simulink model "CluchLockUp"  (R2020b)
settings: Solver=VariableStepAuto  StartTime=0.0  StopTime=10.0  RelTol=1e-3
model workspace (MAT data in the model file):
  Fn = [0  0; 1  0.8; 2  1.6; 3  1.6; 4  1.6; 5  1.6; 6  0.8; 7  0; 8  0; 9  0; 10  0]
  Ie = 1
  Iv = 5
  R = 1
  Tin = [1  2; 2  2; 3  2; 4  2; 5  2; 6  0; 7  0; 8  0; 9  0; 10  0]
  be = 2
  bv = 1
  f1 = [1; 6; 11; 16; 21; 26; 31; 36; 41; 46; 51]
  muk = 1
  mus = 1.5
settings Model: Creator=baner  LastModifiedBy=baner

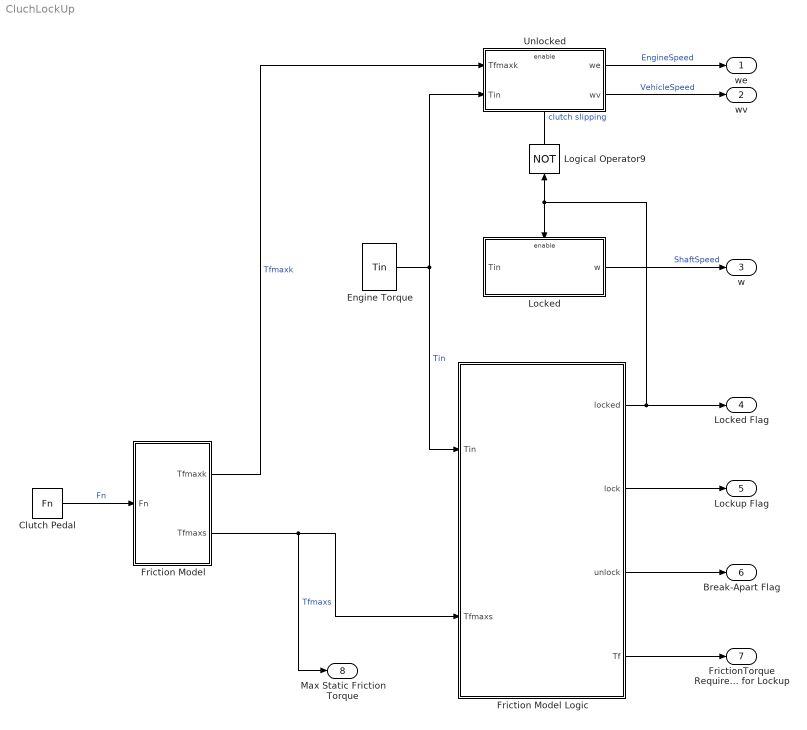
== system CluchLockUp ==
  Clutch Pedal : FromWorkspace  VariableName=Fn  ZeroCross=off
  Engine Torque : FromWorkspace  VariableName=Tin  ZeroCross=off
  Friction Model : Subsystem
  Friction Model Logic : Subsystem
  Locked : Subsystem  TreatAsAtomicUnit=on
  Logical Operator9 : Logic  Operator=NOT  Inputs=1  IconShape=distinctive  OutDataTypeStr=boolean
  Unlocked : Subsystem  TreatAsAtomicUnit=on
  we : Outport  InitialOutput=0  VectorParamsAs1DForOutWhenUnconnected=off
  wv : Outport  Port=2  InitialOutput=0  VectorParamsAs1DForOutWhenUnconnected=off
  w : Outport  Port=3  InitialOutput=0  VectorParamsAs1DForOutWhenUnconnected=off
  Locked Flag : Outport  Port=4  InitialOutput=0  VectorParamsAs1DForOutWhenUnconnected=off
  Lockup Flag : Outport  Port=5  InitialOutput=0  VectorParamsAs1DForOutWhenUnconnected=off
  Break-Apart Flag : Outport  Port=6  InitialOutput=0  VectorParamsAs1DForOutWhenUnconnected=off
  FrictionTorque Required for Lockup : Outport  Port=7  InitialOutput=0  VectorParamsAs1DForOutWhenUnconnected=off
  Max Static Friction Torque : Outport  Port=8  InitialOutput=0  VectorParamsAs1DForOutWhenUnconnected=off
  wires:
  Clutch Pedal/1 -> Friction Model/1(Fn)  "Fn"
  Logical Operator9/1 -> Unlocked/Enable  "clutch slipping"
  Friction Model Logic/1(locked) -> Logical Operator9/1, Locked/Enable, Locked Flag/1
  Engine Torque/1 -> Friction Model Logic/1(Tin), Unlocked/2(Tin)  "Tin"
  Friction Model/1(Tfmaxk) -> Unlocked/1(Tfmaxk)  "Tfmaxk"
  Friction Model/2(Tfmaxs) -> Max Static Friction Torque/1, Friction Model Logic/2(Tfmaxs)  "Tfmaxs"
  Unlocked/1(we) -> we/1  "EngineSpeed"
  Unlocked/2(wv) -> wv/1  "VehicleSpeed"
  Locked/1(w) -> w/1  "ShaftSpeed"
  Friction Model Logic/2(lock) -> Lockup Flag/1
  Friction Model Logic/3(unlock) -> Break-Apart Flag/1
  Friction Model Logic/4(Tf) -> FrictionTorque Required for Lockup/1

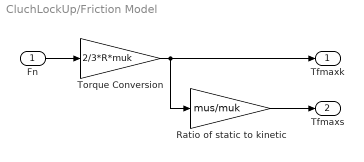
== system CluchLockUp/Friction Model ==
  Fn : Inport
  Ratio of static to kinetic : Gain  Gain=mus/muk  SaturateOnIntegerOverflow=on  OutDataTypeStr=Inherit: Same as input  ParamDataTypeStr=Inherit: Same as input
  Torque Conversion : Gain  Gain=2/3*R*muk  SaturateOnIntegerOverflow=on  OutDataTypeStr=Inherit: Same as input  ParamDataTypeStr=Inherit: Same as input
  Tfmaxk : Outport  InitialOutput=0  VectorParamsAs1DForOutWhenUnconnected=off
  Tfmaxs : Outport  Port=2  InitialOutput=0  VectorParamsAs1DForOutWhenUnconnected=off
  wires:
  Ratio of static to kinetic/1 -> Tfmaxs/1
  Fn/1 -> Torque Conversion/1
  Torque Conversion/1 -> Ratio of static to kinetic/1, Tfmaxk/1

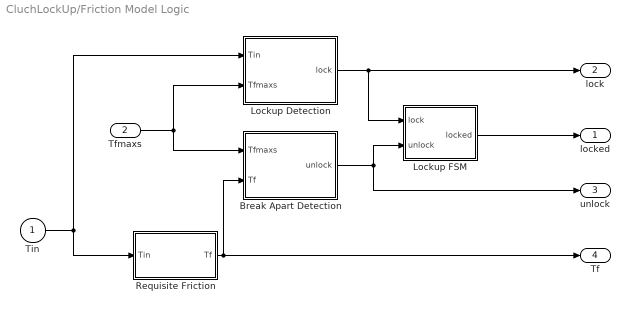
== system CluchLockUp/Friction Model Logic ==
  Tin : Inport
  Tfmaxs : Inport  Port=2
  Break Apart Detection : Subsystem
  Lockup Detection : Subsystem
  Lockup FSM : Subsystem
  Requisite Friction : Subsystem
  locked : Outport  InitialOutput=0  VectorParamsAs1DForOutWhenUnconnected=off
  lock : Outport  Port=2  InitialOutput=0  VectorParamsAs1DForOutWhenUnconnected=off
  unlock : Outport  Port=3  InitialOutput=0  VectorParamsAs1DForOutWhenUnconnected=off
  Tf : Outport  Port=4  InitialOutput=0  VectorParamsAs1DForOutWhenUnconnected=off
  wires:
  Tfmaxs/1 -> Break Apart Detection/1(Tfmaxs), Lockup Detection/2(Tfmaxs)
  Tin/1 -> Requisite Friction/1(Tin), Lockup Detection/1(Tin)
  Requisite Friction/1(Tf) -> Tf/1, Break Apart Detection/2(Tf)
  Lockup Detection/1(lock) -> Lockup FSM/1(lock), lock/1
  Break Apart Detection/1(unlock) -> unlock/1, Lockup FSM/2(unlock)
  Lockup FSM/1(locked) -> locked/1

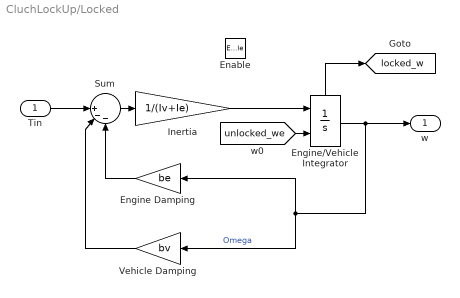
== system CluchLockUp/Locked ==
  Tin : Inport
  Enable : EnablePort  StatesWhenEnabling=reset
  Engine Damping : Gain  Gain=be  SaturateOnIntegerOverflow=on  OutDataTypeStr=Inherit: Same as input  ParamDataTypeStr=Inherit: Same as input
  Engine/Vehicle Integrator : Integrator  InitialConditionSource=external  ShowStatePort=on
  Inertia : Gain  Gain=1/(Iv+Ie)  SaturateOnIntegerOverflow=on  OutDataTypeStr=Inherit: Same as input  ParamDataTypeStr=Inherit: Same as input
  Sum : Sum  Inputs=||+--  InputSameDT=on  SaturateOnIntegerOverflow=on  OutDataTypeStr=Inherit: Same as first input
  Vehicle Damping : Gain  Gain=bv  SaturateOnIntegerOverflow=on  OutDataTypeStr=Inherit: Same as input  ParamDataTypeStr=Inherit: Same as input
  w : Outport  InitialOutput=0  VectorParamsAs1DForOutWhenUnconnected=off
  tag scope: locked_w=global
  wires:
  Vehicle Damping/1 -> Sum/2
  Inertia/1 -> Engine/Vehicle Integrator/1
  Engine Damping/1 -> Sum/3
  Engine/Vehicle Integrator/1 -> Vehicle Damping/1, Engine Damping/1, w/1  "Omega"
  Tin/1 -> Sum/1
  Sum/1 -> Inertia/1
  Engine/Vehicle Integrator/State -> [locked_w]
  [unlocked_we] -> Engine/Vehicle Integrator/2

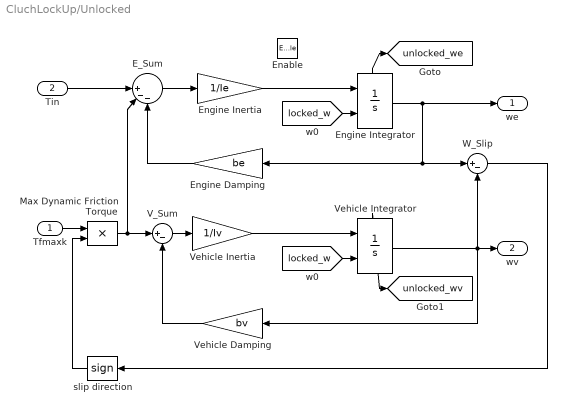
== system CluchLockUp/Unlocked ==
  Tfmaxk : Inport
  Tin : Inport  Port=2
  Enable : EnablePort  StatesWhenEnabling=reset
  E_Sum : Sum  Inputs=||+--  InputSameDT=on  SaturateOnIntegerOverflow=on  OutDataTypeStr=Inherit: Same as first input
  Engine Damping : Gain  Gain=be  SaturateOnIntegerOverflow=on  OutDataTypeStr=Inherit: Same as input  ParamDataTypeStr=Inherit: Same as input
  Engine Inertia : Gain  Gain=1/Ie  SaturateOnIntegerOverflow=on  OutDataTypeStr=Inherit: Same as input  ParamDataTypeStr=Inherit: Same as input
  Engine Integrator : Integrator  InitialConditionSource=external  ShowStatePort=on
  Max Dynamic Friction Torque : Product  InputSameDT=on  RndMeth=Zero  SaturateOnIntegerOverflow=on  OutDataTypeStr=Inherit: Same as first input
  V_Sum : Sum  Inputs=|+-  InputSameDT=on  SaturateOnIntegerOverflow=on  OutDataTypeStr=Inherit: Same as first input
  Vehicle Damping : Gain  Gain=bv  SaturateOnIntegerOverflow=on  OutDataTypeStr=Inherit: Same as input  ParamDataTypeStr=Inherit: Same as input
  Vehicle Inertia : Gain  Gain=1/Iv  SaturateOnIntegerOverflow=on  OutDataTypeStr=Inherit: Same as input  ParamDataTypeStr=Inherit: Same as input
  Vehicle Integrator : Integrator  InitialConditionSource=external  ShowStatePort=on
  W_Slip : Sum  Inputs=|+-  InputSameDT=on  SaturateOnIntegerOverflow=on  OutDataTypeStr=Inherit: Same as first input
  slip direction : Signum
  we : Outport  InitialOutput=0  VectorParamsAs1DForOutWhenUnconnected=off
  wv : Outport  Port=2  InitialOutput=0  VectorParamsAs1DForOutWhenUnconnected=off
  tag scope: unlocked_we=global, unlocked_wv=global
  wires:
  Vehicle Integrator/1 -> Vehicle Damping/1, W_Slip/2, wv/1
  Vehicle Inertia/1 -> Vehicle Integrator/1
  [locked_w] -> Vehicle Integrator/2
  Vehicle Integrator/State -> [unlocked_wv]
  Tin/1 -> E_Sum/1
  [locked_w] -> Engine Integrator/2
  Engine Integrator/1 -> W_Slip/1, Engine Damping/1, we/1
  Engine Damping/1 -> E_Sum/3
  E_Sum/1 -> Engine Inertia/1
  Engine Inertia/1 -> Engine Integrator/1
  Engine Integrator/State -> [unlocked_we]
  W_Slip/1 -> slip direction/1
  slip direction/1 -> Max Dynamic Friction Torque/2
  Tfmaxk/1 -> Max Dynamic Friction Torque/1
  Max Dynamic Friction Torque/1 -> E_Sum/2, V_Sum/1
  Vehicle Damping/1 -> V_Sum/2
  V_Sum/1 -> Vehicle Inertia/1

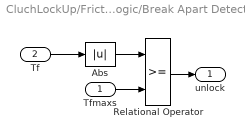
== system CluchLockUp/Friction Model Logic/Break Apart Detection ==
  Tfmaxs : Inport
  Tf : Inport  Port=2
  Abs : Abs  SaturateOnIntegerOverflow=on
  Relational Operator : RelationalOperator  OutDataTypeStr=boolean  RndMeth=Nearest  InputSameDT=on
  unlock : Outport  InitialOutput=0  VectorParamsAs1DForOutWhenUnconnected=off
  wires:
  Tfmaxs/1 -> Relational Operator/2
  Abs/1 -> Relational Operator/1
  Relational Operator/1 -> unlock/1
  Tf/1 -> Abs/1

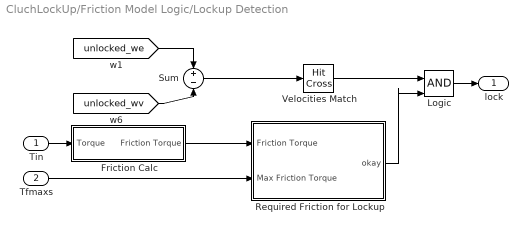
== system CluchLockUp/Friction Model Logic/Lockup Detection ==
  Tin : Inport
  Tfmaxs : Inport  Port=2
  Friction Calc : Subsystem
  Logic : Logic  IconShape=distinctive  OutDataTypeStr=boolean
  Required Friction for Lockup : Subsystem
  Sum : Sum  Inputs=+-  InputSameDT=on  SaturateOnIntegerOverflow=on  OutDataTypeStr=Inherit: Same as first input
  Velocities Match : HitCross
  lock : Outport  InitialOutput=0  VectorParamsAs1DForOutWhenUnconnected=off
  wires:
  Tin/1 -> Friction Calc/1(Torque)
  Sum/1 -> Velocities Match/1
  [unlocked_wv] -> Sum/2
  [unlocked_we] -> Sum/1
  Required Friction for Lockup/1(okay) -> Logic/2
  Logic/1 -> lock/1
  Velocities Match/1 -> Logic/1
  Tfmaxs/1 -> Required Friction for Lockup/2(Max Friction Torque)
  Friction Calc/1(Friction Torque) -> Required Friction for Lockup/1(Friction Torque)

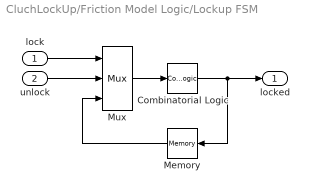
== system CluchLockUp/Friction Model Logic/Lockup FSM ==
  lock : Inport
  unlock : Inport  Port=2
  Combinatorial Logic : CombinatorialLogic  TruthTable=[0;1;0;0;1;1;1;0]
  Memory : Memory
  Mux : Mux  Inputs=3
  locked : Outport  InitialOutput=0  VectorParamsAs1DForOutWhenUnconnected=off
  wires:
  Mux/1 -> Combinatorial Logic/1
  lock/1 -> Mux/1
  unlock/1 -> Mux/2
  Combinatorial Logic/1 -> Memory/1, locked/1
  Memory/1 -> Mux/3

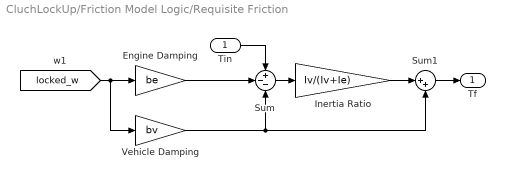
== system CluchLockUp/Friction Model Logic/Requisite Friction ==
  Tin : Inport
  Engine Damping : Gain  Gain=be  SaturateOnIntegerOverflow=on  OutDataTypeStr=Inherit: Same as input  ParamDataTypeStr=Inherit: Same as input
  Inertia Ratio : Gain  Gain=Iv/(Iv+Ie)  SaturateOnIntegerOverflow=on  OutDataTypeStr=Inherit: Same as input  ParamDataTypeStr=Inherit: Same as input
  Sum : Sum  Inputs=+--  InputSameDT=on  SaturateOnIntegerOverflow=on  OutDataTypeStr=Inherit: Same as first input
  Sum1 : Sum  Inputs=|++  InputSameDT=on  SaturateOnIntegerOverflow=on  OutDataTypeStr=Inherit: Same as first input
  Vehicle Damping : Gain  Gain=bv  SaturateOnIntegerOverflow=on  OutDataTypeStr=Inherit: Same as input  ParamDataTypeStr=Inherit: Same as input
  Tf : Outport  InitialOutput=0  VectorParamsAs1DForOutWhenUnconnected=off
  wires:
  Sum1/1 -> Tf/1
  Inertia Ratio/1 -> Sum1/1
  Tin/1 -> Sum/1
  Sum/1 -> Inertia Ratio/1
  Vehicle Damping/1 -> Sum1/2, Sum/3
  Engine Damping/1 -> Sum/2
  [locked_w] -> Engine Damping/1, Vehicle Damping/1

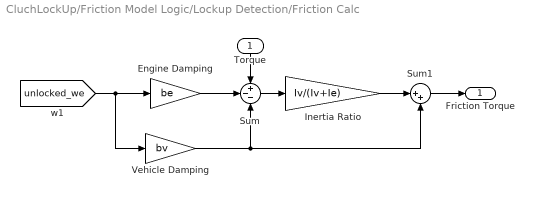
== system CluchLockUp/Friction Model Logic/Lockup Detection/Friction Calc ==
  Torque : Inport
  Engine Damping : Gain  Gain=be  SaturateOnIntegerOverflow=on  OutDataTypeStr=Inherit: Same as input  ParamDataTypeStr=Inherit: Same as input
  Inertia Ratio : Gain  Gain=Iv/(Iv+Ie)  SaturateOnIntegerOverflow=on  OutDataTypeStr=Inherit: Same as input  ParamDataTypeStr=Inherit: Same as input
  Sum : Sum  Inputs=+--  InputSameDT=on  SaturateOnIntegerOverflow=on  OutDataTypeStr=Inherit: Same as first input
  Sum1 : Sum  Inputs=|++  InputSameDT=on  SaturateOnIntegerOverflow=on  OutDataTypeStr=Inherit: Same as first input
  Vehicle Damping : Gain  Gain=bv  SaturateOnIntegerOverflow=on  OutDataTypeStr=Inherit: Same as input  ParamDataTypeStr=Inherit: Same as input
  Friction Torque : Outport  InitialOutput=0  VectorParamsAs1DForOutWhenUnconnected=off
  wires:
  Sum1/1 -> Friction Torque/1
  Inertia Ratio/1 -> Sum1/1
  Torque/1 -> Sum/1
  Sum/1 -> Inertia Ratio/1
  Engine Damping/1 -> Sum/2
  Vehicle Damping/1 -> Sum/3, Sum1/2
  [unlocked_we] -> Vehicle Damping/1, Engine Damping/1

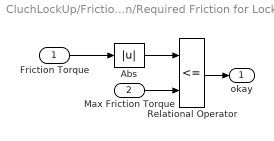
== system CluchLockUp/Friction Model Logic/Lockup Detection/Required Friction for Lockup ==
  Friction Torque : Inport
  Max Friction Torque : Inport  Port=2
  Abs : Abs  SaturateOnIntegerOverflow=on
  Relational Operator : RelationalOperator  Operator=<=  OutDataTypeStr=boolean  RndMeth=Nearest  InputSameDT=on
  okay : Outport  InitialOutput=0  VectorParamsAs1DForOutWhenUnconnected=off
  wires:
  Max Friction Torque/1 -> Relational Operator/2
  Abs/1 -> Relational Operator/1
  Relational Operator/1 -> okay/1
  Friction Torque/1 -> Abs/1
